simulink model "QZhLBPID"  (Simulink 5.0)
settings: Solver=ode4  StartTime=0.0  StopTime=8000  FixedStep=20  RelTol=1e-3
settings Model: LastModifiedBy=ThinkPad

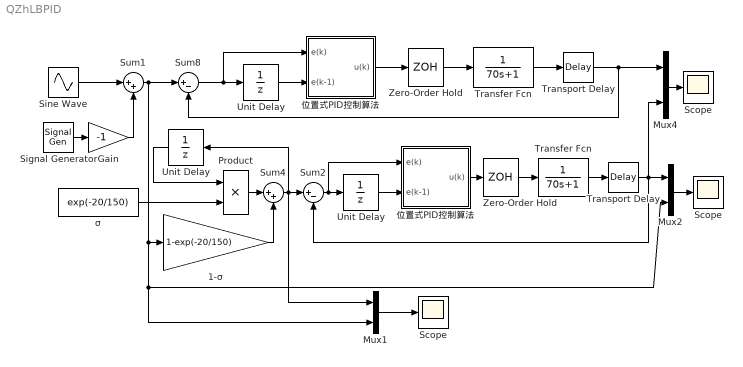
== system QZhLBPID ==
  " Scope " : Scope
      settings: YMin=-1.2  YMax=1.2  SaveName=QZhLBPID  DataFormat=Array  MaxDataPoints=500000
  " Unit Delay " : UnitDelay  Orientation=left  SampleTime=20
  " 位置式PID控制算法 " : Subsystem
  1-σ : Gain  Gain=1-exp(-20/150)  SaturateOnIntegerOverflow=on
  Gain : Gain  Gain=-1  SaturateOnIntegerOverflow=on
  Mux1 : Mux  Inputs=2
  Mux2 : Mux  Inputs=2
  Mux4 : Mux  Inputs=2
  "Product " : Product  SaturateOnIntegerOverflow=on
  Scope : Scope
      settings: YMin=-1.2  YMax=1.2  SaveName=QZhLBPIDPID  DataFormat=Array  MaxDataPoints=500000
  "Scope  " : Scope
      settings: YMin=-1.2  YMax=1.2  SaveName=QZhLBPIDry  DataFormat=Array  MaxDataPoints=500000
  "Signal Generator " : SignalGenerator  WaveForm=square  Frequency=0.0005*pi  Units=rad/sec
  "Sine Wave " : Sin  Amplitude=0.05  Frequency=0.03*pi  SampleTime=0
  Sum1 : Sum  Inputs=|++  SaturateOnIntegerOverflow=on
  Sum2 : Sum  Inputs=|+-  SaturateOnIntegerOverflow=on
  Sum4 : Sum  Inputs=|++  SaturateOnIntegerOverflow=on
  Sum8 : Sum  Inputs=|+-  SaturateOnIntegerOverflow=on
  Transfer Fcn : TransferFcn  Denominator=[70 1]
  "Transfer Fcn " : TransferFcn  Denominator=[70 1]
  Transport Delay : TransportDelay  DelayTime=80
  "Transport Delay " : TransportDelay  DelayTime=80
  Unit Delay : UnitDelay  SampleTime=20
  "Unit Delay " : UnitDelay  SampleTime=20
  Zero-Order Hold : ZeroOrderHold  SampleTime=20
  "Zero-Order Hold " : ZeroOrderHold  SampleTime=20
  σ : Constant  Value=exp(-20/150)
  "位置式PID控制算法 " : Subsystem
  wires:
  Sum1/1 -> 1-σ/1, Mux2/2, Mux1/2, Sum8/1
  Transfer Fcn/1 -> Transport Delay/1
  " 位置式PID控制算法 "/1(u(k)) -> Zero-Order Hold/1
  Sum8/1 -> Unit Delay/1, " 位置式PID控制算法 "/1(e(k))
  Zero-Order Hold/1 -> Transfer Fcn/1
  Mux4/1 -> Scope/1
  Transport Delay/1 -> Sum8/2, Mux4/1
  Unit Delay/1 -> " 位置式PID控制算法 "/2(e(k-1))
  "Transfer Fcn "/1 -> "Transport Delay "/1
  "位置式PID控制算法 "/1(u(k)) -> "Zero-Order Hold "/1
  Sum2/1 -> "Unit Delay "/1, "位置式PID控制算法 "/1(e(k))
  "Zero-Order Hold "/1 -> "Transfer Fcn "/1
  Mux2/1 -> "Scope  "/1
  "Transport Delay "/1 -> Mux2/1, Mux4/2, Sum2/2
  "Unit Delay "/1 -> "位置式PID控制算法 "/2(e(k-1))
  "Product "/1 -> Sum4/1
  σ/1 -> "Product "/2
  Sum4/1 -> " Unit Delay "/1, Mux1/1, Sum2/1
  " Unit Delay "/1 -> "Product "/1
  "Sine Wave "/1 -> Sum1/1
  "Signal Generator "/1 -> Gain/1
  Gain/1 -> Sum1/2
  1-σ/1 -> Sum4/2
  Mux1/1 -> " Scope "/1

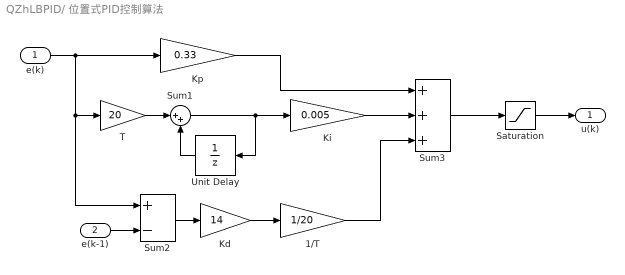
== system QZhLBPID/ 位置式PID控制算法  ==
  e(k) : Inport
  e(k-1) : Inport  Port=2
  1/T : Gain  Gain=1/20  SaturateOnIntegerOverflow=on
  Kd : Gain  Gain=14  SaturateOnIntegerOverflow=on
  Ki : Gain  Gain=0.005  SaturateOnIntegerOverflow=on
  Kp : Gain  Gain=0.33  SaturateOnIntegerOverflow=on
  Saturation : Saturate  UpperLimit=10  LowerLimit=-10
  Sum1 : Sum  Inputs=|++  SaturateOnIntegerOverflow=on
  Sum2 : Sum  Inputs=+-  SaturateOnIntegerOverflow=on
  Sum3 : Sum  Inputs=+++  SaturateOnIntegerOverflow=on
  T : Gain  Gain=20  SaturateOnIntegerOverflow=on
  "Unit Delay " : UnitDelay  Orientation=left  SampleTime=20
  u(k) : Outport
  wires:
  T/1 -> Sum1/1
  Sum2/1 -> Kd/1
  e(k)/1 -> Kp/1, Sum2/1, T/1
  Kp/1 -> Sum3/1
  Ki/1 -> Sum3/2
  Sum3/1 -> Saturation/1
  Saturation/1 -> u(k)/1
  Kd/1 -> 1/T/1
  e(k-1)/1 -> Sum2/2
  1/T/1 -> Sum3/3
  Sum1/1 -> "Unit Delay "/1, Ki/1
  "Unit Delay "/1 -> Sum1/2

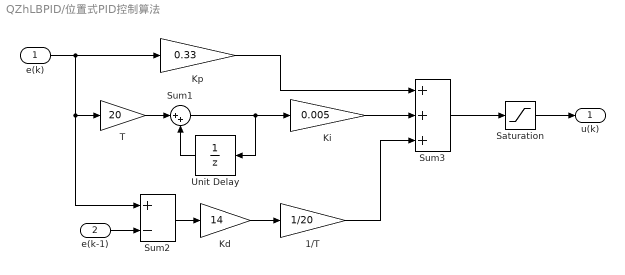
== system QZhLBPID/位置式PID控制算法  ==
  e(k) : Inport
  e(k-1) : Inport  Port=2
  1/T : Gain  Gain=1/20  SaturateOnIntegerOverflow=on
  Kd : Gain  Gain=14  SaturateOnIntegerOverflow=on
  Ki : Gain  Gain=0.005  SaturateOnIntegerOverflow=on
  Kp : Gain  Gain=0.33  SaturateOnIntegerOverflow=on
  Saturation : Saturate  UpperLimit=10  LowerLimit=-10
  Sum1 : Sum  Inputs=|++  SaturateOnIntegerOverflow=on
  Sum2 : Sum  Inputs=+-  SaturateOnIntegerOverflow=on
  Sum3 : Sum  Inputs=+++  SaturateOnIntegerOverflow=on
  T : Gain  Gain=20  SaturateOnIntegerOverflow=on
  "Unit Delay " : UnitDelay  Orientation=left  SampleTime=20
  u(k) : Outport
  wires:
  T/1 -> Sum1/1
  Sum2/1 -> Kd/1
  e(k)/1 -> Kp/1, Sum2/1, T/1
  Kp/1 -> Sum3/1
  Ki/1 -> Sum3/2
  Sum3/1 -> Saturation/1
  Saturation/1 -> u(k)/1
  Kd/1 -> 1/T/1
  e(k-1)/1 -> Sum2/2
  1/T/1 -> Sum3/3
  Sum1/1 -> "Unit Delay "/1, Ki/1
  "Unit Delay "/1 -> Sum1/2
